simulink library "LibDBC_Some_Node_ch0_ORIGINAL"  (Simulink 9.1)
settings: Solver=VariableStepAuto  StartTime=0.0  StopTime=10.0  RelTol=1e-3
undefined symbols (not defined in the file): bit_packing, bit_unpacking, IO_Blk_Lib_TTC500, IO_CAN_ConfigMsg
libraries: IOBlock_Library_TTC580 x4, simulink x2
(part 1 of 2)
Description:
  | 10-Mai-2016 10:50:501823
settings Model: Creator=hokka  LastModifiedBy=hokka

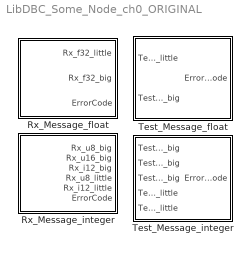
== system LibDBC_Some_Node_ch0_ORIGINAL ==
  Rx_Message_float : Subsystem  Priority=0
  Rx_Message_integer : Subsystem  Priority=0
  Test_Message_float : Subsystem  Priority=0
  Test_Message_integer : Subsystem  Priority=0

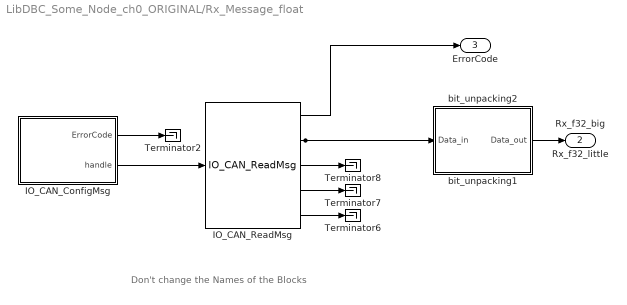
== system LibDBC_Some_Node_ch0_ORIGINAL/Rx_Message_float ==
  note: Don't change the Names of the Blocks
  IO_CAN_ConfigMsg : Subsystem  mask(IO_CAN_ConfigMsg_Code){SampleTime=-1, ttlib=IO_Blk_Lib_TTC500, ttDescription=IO_CAN_ConfigMsg, tt_iolib_version=0.19, channel=IO_CAN_CHANNEL_0, mode=IO_CAN_MSG_READ, id_format=IO_CAN_EXT_FRAME, id=0x00001021, ac_mask=0x1FFFFFFF}
      mask help: Configures a message object for the given CAN channel.
      mask init:
      | %
      mask Help: web(which('IO_CAN.h'))
      mask TypeOptions channel: IO_CAN_CHANNEL_0  | IO_CAN_CHANNEL_1 | IO_CAN_CHANNEL_2 | IO_CAN_CHANNEL_3 | IO_CAN_CHANNEL_4 | IO_CAN_CHANNEL_5 | IO_CAN_CHANNEL_6
      mask Callback channel: %
      mask TypeOptions mode: IO_CAN_MSG_READ | IO_CAN_MSG_WRITE
      mask Callback mode: %
      mask TypeOptions id_format: IO_CAN_STD_FRAME | IO_CAN_EXT_FRAME
      mask Callback id_format: %
      mask Callback id: %
      mask Callback ac_mask: %
  IO_CAN_ReadMsg : IOBlock_Library_TTC580/CAN  Blocks TTC580 IOlib/ReadMsg_CAN/IO_CAN_ReadMsg  SampleTime=-1  ttlib=IO_Blk_Lib_TTC500  ttDescription=IO_CAN_ReadMsg  tt_iolib_version=0.19
      settings: SourceProductName=I/O Blocklibrary for TTC580
  Terminator{2,6..8} (4 alike) : Terminator
  bit_unpacking1 : Subsystem  LoadFcn=|  mask(bit_unpacking_Code){SampleTime=-1, ttlib=IO_Blk_Lib_TTC500, ttDescription=bit_unpacking, tt_iolib_version=0.19, Endianness=little, Format=real32, Inversion=off, Startbit=0, Width_bits=32, Factor=1, Offset=0}
      | try
      | %
      | %Upgrade Information - standard BEGIN
      | new_color = 'blue';
      | new_ver = '0.19';
      | act_ver = get_param(gcb,'tt_iolib_version');
      | if not(strcmp(act_ver,new_ver))
      |     disp(['Upgrade block: ',gcb,char(10),'       Version: ',act_ver,' -> ',new_ver]);
      |     %switch - case for specific upgrade information e.g. additional parameter required 
      |     %Change appearance and version information
      |     set_param(gcb,'ForegroundColor',new_color);
      |     set_param(gcb,'tt_iolib_version',new_ver);
      | end
      | %Upgrade Information - standard END
      | catch
      | %Standard catch section BEGIN 
      | disp(' ');
      | disp('------------------------------------------------------------');
      | disp('An error occurred in a callback of the TTC580-BlockLib.');
      | disp(['Please check the parameters in the mask of ',gcb]);
      | disp('If you do not encounter any violations, then please '); 
      | disp('copy the following lines and report this to support@ttcontrol.com ');
      | disp('<< begin of error message dump >>');
      | disp(['Version of TTC580-BlockLib: ', get_param(gcb,'tt_iolib_version')]);
      | disp(get_param(gcb,'ttDescription'));
      | disp(gcb);
      | x=lasterror;disp(x.message);
      | disp(get_param(gcb,'MaskValues'));
      | disp(version);
      | disp(computer);
      | disp('<< end of error message dump >>');
      | disp('------------------------------------------------------------');
      | disp(' ');
      | %Standard catch section END
      | end
      mask help:
      | Block to read in CAN signal from a specified position within 64bit field.
      | For "Factor" and "Offset" the definition of Vector's CANdb applies:
      | [Physical value] = ( [Raw value] * [Factor] ) + [Offset]
      | with Raw value of a signal being the value as it is transmitted in the CAN-network
      mask init:
      | %
      mask Help: web(which('IOLib500_utils.h'))
      mask TypeOptions Endianness: big | little
      mask Callback Endianness: %
      mask TypeOptions Format: unsigned | signed | real32
      mask Callback Format: %
      mask Callback Inversion: %
      mask Callback Startbit: %
      mask Callback Width_bits: %
      mask Callback Factor: %
      mask Callback Offset: %
  bit_unpacking2 : Subsystem  LoadFcn=|  mask(bit_unpacking_Code){SampleTime=-1, ttlib=IO_Blk_Lib_TTC500, ttDescription=bit_unpacking, tt_iolib_version=0.19, Endianness=big, Format=real32, Inversion=off, Startbit=56, Width_bits=32, Factor=1, Offset=0}
      | try
      | %
      | %Upgrade Information - standard BEGIN
      | new_color = 'blue';
      | new_ver = '0.19';
      | act_ver = get_param(gcb,'tt_iolib_version');
      | if not(strcmp(act_ver,new_ver))
      |     disp(['Upgrade block: ',gcb,char(10),'       Version: ',act_ver,' -> ',new_ver]);
      |     %switch - case for specific upgrade information e.g. additional parameter required 
      |     %Change appearance and version information
      |     set_param(gcb,'ForegroundColor',new_color);
      |     set_param(gcb,'tt_iolib_version',new_ver);
      | end
      | %Upgrade Information - standard END
      | catch
      | %Standard catch section BEGIN 
      | disp(' ');
      | disp('------------------------------------------------------------');
      | disp('An error occurred in a callback of the TTC580-BlockLib.');
      | disp(['Please check the parameters in the mask of ',gcb]);
      | disp('If you do not encounter any violations, then please '); 
      | disp('copy the following lines and report this to support@ttcontrol.com ');
      | disp('<< begin of error message dump >>');
      | disp(['Version of TTC580-BlockLib: ', get_param(gcb,'tt_iolib_version')]);
      | disp(get_param(gcb,'ttDescription'));
      | disp(gcb);
      | x=lasterror;disp(x.message);
      | disp(get_param(gcb,'MaskValues'));
      | disp(version);
      | disp(computer);
      | disp('<< end of error message dump >>');
      | disp('------------------------------------------------------------');
      | disp(' ');
      | %Standard catch section END
      | end
      mask help:
      | Block to read in CAN signal from a specified position within 64bit field.
      | For "Factor" and "Offset" the definition of Vector's CANdb applies:
      | [Physical value] = ( [Raw value] * [Factor] ) + [Offset]
      | with Raw value of a signal being the value as it is transmitted in the CAN-network
      mask init:
      | %
      mask Help: web(which('IOLib500_utils.h'))
      mask TypeOptions Endianness: big | little
      mask Callback Endianness: %
      mask TypeOptions Format: unsigned | signed | real32
      mask Callback Format: %
      mask Callback Inversion: %
      mask Callback Startbit: %
      mask Callback Width_bits: %
      mask Callback Factor: %
      mask Callback Offset: %
  Rx_f32_little : Outport
  Rx_f32_big : Outport  Port=2
  ErrorCode : Outport  Port=3
  wires:
  IO_CAN_ReadMsg/3 -> Terminator8/1
  IO_CAN_ReadMsg/4 -> Terminator7/1
  IO_CAN_ReadMsg/5 -> Terminator6/1
  IO_CAN_ConfigMsg/2(handle) -> IO_CAN_ReadMsg/1
  IO_CAN_ConfigMsg/1(ErrorCode) -> Terminator2/1
  IO_CAN_ReadMsg/1 -> ErrorCode/1
  IO_CAN_ReadMsg/2 -> bit_unpacking1/1(Data_in), bit_unpacking2/1(Data_in)
  bit_unpacking1/1(Data_out) -> Rx_f32_little/1
  bit_unpacking2/1(Data_out) -> Rx_f32_big/1

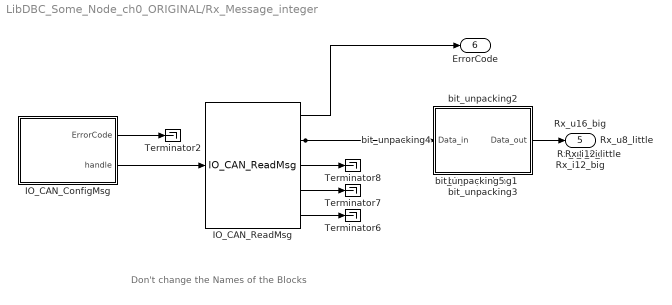
== system LibDBC_Some_Node_ch0_ORIGINAL/Rx_Message_integer ==
  note: Don't change the Names of the Blocks
  IO_CAN_ConfigMsg : Subsystem  mask(IO_CAN_ConfigMsg_Code){SampleTime=-1, ttlib=IO_Blk_Lib_TTC500, ttDescription=IO_CAN_ConfigMsg, tt_iolib_version=0.19, channel=IO_CAN_CHANNEL_0, mode=IO_CAN_MSG_READ, id_format=IO_CAN_STD_FRAME, id=0x020, ac_mask=0x7FF}
      mask help: Configures a message object for the given CAN channel.
      mask init:
      | %
      mask Help: web(which('IO_CAN.h'))
      mask TypeOptions channel: IO_CAN_CHANNEL_0  | IO_CAN_CHANNEL_1 | IO_CAN_CHANNEL_2 | IO_CAN_CHANNEL_3 | IO_CAN_CHANNEL_4 | IO_CAN_CHANNEL_5 | IO_CAN_CHANNEL_6
      mask Callback channel: %
      mask TypeOptions mode: IO_CAN_MSG_READ | IO_CAN_MSG_WRITE
      mask Callback mode: %
      mask TypeOptions id_format: IO_CAN_STD_FRAME | IO_CAN_EXT_FRAME
      mask Callback id_format: %
      mask Callback id: %
      mask Callback ac_mask: %
  IO_CAN_ReadMsg : IOBlock_Library_TTC580/CAN  Blocks TTC580 IOlib/ReadMsg_CAN/IO_CAN_ReadMsg  SampleTime=-1  ttlib=IO_Blk_Lib_TTC500  ttDescription=IO_CAN_ReadMsg  tt_iolib_version=0.19
      settings: SourceProductName=I/O Blocklibrary for TTC580
  Terminator{2,6..8} (4 alike) : Terminator
  bit_unpacking1 : Subsystem  LoadFcn=|  mask(bit_unpacking_Code){SampleTime=-1, ttlib=IO_Blk_Lib_TTC500, ttDescription=bit_unpacking, tt_iolib_version=0.19, Endianness=big, Format=unsigned, Inversion=off, Startbit=0, Width_bits=8, Factor=1, Offset=0}
      | try
      | %
      | %Upgrade Information - standard BEGIN
      | new_color = 'blue';
      | new_ver = '0.19';
      | act_ver = get_param(gcb,'tt_iolib_version');
      | if not(strcmp(act_ver,new_ver))
      |     disp(['Upgrade block: ',gcb,char(10),'       Version: ',act_ver,' -> ',new_ver]);
      |     %switch - case for specific upgrade information e.g. additional parameter required 
      |     %Change appearance and version information
      |     set_param(gcb,'ForegroundColor',new_color);
      |     set_param(gcb,'tt_iolib_version',new_ver);
      | end
      | %Upgrade Information - standard END
      | catch
      | %Standard catch section BEGIN 
      | disp(' ');
      | disp('------------------------------------------------------------');
      | disp('An error occurred in a callback of the TTC580-BlockLib.');
      | disp(['Please check the parameters in the mask of ',gcb]);
      | disp('If you do not encounter any violations, then please '); 
      | disp('copy the following lines and report this to support@ttcontrol.com ');
      | disp('<< begin of error message dump >>');
      | disp(['Version of TTC580-BlockLib: ', get_param(gcb,'tt_iolib_version')]);
      | disp(get_param(gcb,'ttDescription'));
      | disp(gcb);
      | x=lasterror;disp(x.message);
      | disp(get_param(gcb,'MaskValues'));
      | disp(version);
      | disp(computer);
      | disp('<< end of error message dump >>');
      | disp('------------------------------------------------------------');
      | disp(' ');
      | %Standard catch section END
      | end
      mask help:
      | Block to read in CAN signal from a specified position within 64bit field.
      | For "Factor" and "Offset" the definition of Vector's CANdb applies:
      | [Physical value] = ( [Raw value] * [Factor] ) + [Offset]
      | with Raw value of a signal being the value as it is transmitted in the CAN-network
      mask init:
      | %
      mask Help: web(which('IOLib500_utils.h'))
      mask TypeOptions Endianness: big | little
      mask Callback Endianness: %
      mask TypeOptions Format: unsigned | signed | real32
      mask Callback Format: %
      mask Callback Inversion: %
      mask Callback Startbit: %
      mask Callback Width_bits: %
      mask Callback Factor: %
      mask Callback Offset: %
  bit_unpacking2 : Subsystem  LoadFcn=|  mask(bit_unpacking_Code){SampleTime=-1, ttlib=IO_Blk_Lib_TTC500, ttDescription=bit_unpacking, tt_iolib_version=0.19, Endianness=big, Format=unsigned, Inversion=off, Startbit=16, Width_bits=16, Factor=1, Offset=0}
      | try
      | %
      | %Upgrade Information - standard BEGIN
      | new_color = 'blue';
      | new_ver = '0.19';
      | act_ver = get_param(gcb,'tt_iolib_version');
      | if not(strcmp(act_ver,new_ver))
      |     disp(['Upgrade block: ',gcb,char(10),'       Version: ',act_ver,' -> ',new_ver]);
      |     %switch - case for specific upgrade information e.g. additional parameter required 
      |     %Change appearance and version information
      |     set_param(gcb,'ForegroundColor',new_color);
      |     set_param(gcb,'tt_iolib_version',new_ver);
      | end
      | %Upgrade Information - standard END
      | catch
      | %Standard catch section BEGIN 
      | disp(' ');
      | disp('------------------------------------------------------------');
      | disp('An error occurred in a callback of the TTC580-BlockLib.');
      | disp(['Please check the parameters in the mask of ',gcb]);
      | disp('If you do not encounter any violations, then please '); 
      | disp('copy the following lines and report this to support@ttcontrol.com ');
      | disp('<< begin of error message dump >>');
      | disp(['Version of TTC580-BlockLib: ', get_param(gcb,'tt_iolib_version')]);
      | disp(get_param(gcb,'ttDescription'));
      | disp(gcb);
      | x=lasterror;disp(x.message);
      | disp(get_param(gcb,'MaskValues'));
      | disp(version);
      | disp(computer);
      | disp('<< end of error message dump >>');
      | disp('------------------------------------------------------------');
      | disp(' ');
      | %Standard catch section END
      | end
      mask help:
      | Block to read in CAN signal from a specified position within 64bit field.
      | For "Factor" and "Offset" the definition of Vector's CANdb applies:
      | [Physical value] = ( [Raw value] * [Factor] ) + [Offset]
      | with Raw value of a signal being the value as it is transmitted in the CAN-network
      mask init:
      | %
      mask Help: web(which('IOLib500_utils.h'))
      mask TypeOptions Endianness: big | little
      mask Callback Endianness: %
      mask TypeOptions Format: unsigned | signed | real32
      mask Callback Format: %
      mask Callback Inversion: %
      mask Callback Startbit: %
      mask Callback Width_bits: %
      mask Callback Factor: %
      mask Callback Offset: %
  bit_unpacking3 : Subsystem  LoadFcn=|  mask(bit_unpacking_Code){SampleTime=-1, ttlib=IO_Blk_Lib_TTC500, ttDescription=bit_unpacking, tt_iolib_version=0.19, Endianness=big, Format=signed, Inversion=off, Startbit=35, Width_bits=12, Factor=1, Offset=0}
      | try
      | %
      | %Upgrade Information - standard BEGIN
      | new_color = 'blue';
      | new_ver = '0.19';
      | act_ver = get_param(gcb,'tt_iolib_version');
      | if not(strcmp(act_ver,new_ver))
      |     disp(['Upgrade block: ',gcb,char(10),'       Version: ',act_ver,' -> ',new_ver]);
      |     %switch - case for specific upgrade information e.g. additional parameter required 
      |     %Change appearance and version information
      |     set_param(gcb,'ForegroundColor',new_color);
      |     set_param(gcb,'tt_iolib_version',new_ver);
      | end
      | %Upgrade Information - standard END
      | catch
      | %Standard catch section BEGIN 
      | disp(' ');
      | disp('------------------------------------------------------------');
      | disp('An error occurred in a callback of the TTC580-BlockLib.');
      | disp(['Please check the parameters in the mask of ',gcb]);
      | disp('If you do not encounter any violations, then please '); 
      | disp('copy the following lines and report this to support@ttcontrol.com ');
      | disp('<< begin of error message dump >>');
      | disp(['Version of TTC580-BlockLib: ', get_param(gcb,'tt_iolib_version')]);
      | disp(get_param(gcb,'ttDescription'));
      | disp(gcb);
      | x=lasterror;disp(x.message);
      | disp(get_param(gcb,'MaskValues'));
      | disp(version);
      | disp(computer);
      | disp('<< end of error message dump >>');
      | disp('------------------------------------------------------------');
      | disp(' ');
      | %Standard catch section END
      | end
      mask help:
      | Block to read in CAN signal from a specified position within 64bit field.
      | For "Factor" and "Offset" the definition of Vector's CANdb applies:
      | [Physical value] = ( [Raw value] * [Factor] ) + [Offset]
      | with Raw value of a signal being the value as it is transmitted in the CAN-network
      mask init:
      | %
      mask Help: web(which('IOLib500_utils.h'))
      mask TypeOptions Endianness: big | little
      mask Callback Endianness: %
      mask TypeOptions Format: unsigned | signed | real32
      mask Callback Format: %
      mask Callback Inversion: %
      mask Callback Startbit: %
      mask Callback Width_bits: %
      mask Callback Factor: %
      mask Callback Offset: %
  bit_unpacking4 : Subsystem  LoadFcn=|  mask(bit_unpacking_Code){SampleTime=-1, ttlib=IO_Blk_Lib_TTC500, ttDescription=bit_unpacking, tt_iolib_version=0.19, Endianness=little, Format=unsigned, Inversion=off, Startbit=40, Width_bits=8, Factor=1, Offset=0}
      | try
      | %
      | %Upgrade Information - standard BEGIN
      | new_color = 'blue';
      | new_ver = '0.19';
      | act_ver = get_param(gcb,'tt_iolib_version');
      | if not(strcmp(act_ver,new_ver))
      |     disp(['Upgrade block: ',gcb,char(10),'       Version: ',act_ver,' -> ',new_ver]);
      |     %switch - case for specific upgrade information e.g. additional parameter required 
      |     %Change appearance and version information
      |     set_param(gcb,'ForegroundColor',new_color);
      |     set_param(gcb,'tt_iolib_version',new_ver);
      | end
      | %Upgrade Information - standard END
      | catch
      | %Standard catch section BEGIN 
      | disp(' ');
      | disp('------------------------------------------------------------');
      | disp('An error occurred in a callback of the TTC580-BlockLib.');
      | disp(['Please check the parameters in the mask of ',gcb]);
      | disp('If you do not encounter any violations, then please '); 
      | disp('copy the following lines and report this to support@ttcontrol.com ');
      | disp('<< begin of error message dump >>');
      | disp(['Version of TTC580-BlockLib: ', get_param(gcb,'tt_iolib_version')]);
      | disp(get_param(gcb,'ttDescription'));
      | disp(gcb);
      | x=lasterror;disp(x.message);
      | disp(get_param(gcb,'MaskValues'));
      | disp(version);
      | disp(computer);
      | disp('<< end of error message dump >>');
      | disp('------------------------------------------------------------');
      | disp(' ');
      | %Standard catch section END
      | end
      mask help:
      | Block to read in CAN signal from a specified position within 64bit field.
      | For "Factor" and "Offset" the definition of Vector's CANdb applies:
      | [Physical value] = ( [Raw value] * [Factor] ) + [Offset]
      | with Raw value of a signal being the value as it is transmitted in the CAN-network
      mask init:
      | %
      mask Help: web(which('IOLib500_utils.h'))
      mask TypeOptions Endianness: big | little
      mask Callback Endianness: %
      mask TypeOptions Format: unsigned | signed | real32
      mask Callback Format: %
      mask Callback Inversion: %
      mask Callback Startbit: %
      mask Callback Width_bits: %
      mask Callback Factor: %
      mask Callback Offset: %
  bit_unpacking5 : Subsystem  LoadFcn=|  mask(bit_unpacking_Code){SampleTime=-1, ttlib=IO_Blk_Lib_TTC500, ttDescription=bit_unpacking, tt_iolib_version=0.19, Endianness=little, Format=signed, Inversion=off, Startbit=49, Width_bits=12, Factor=1, Offset=0}
      | try
      | %
      | %Upgrade Information - standard BEGIN
      | new_color = 'blue';
      | new_ver = '0.19';
      | act_ver = get_param(gcb,'tt_iolib_version');
      | if not(strcmp(act_ver,new_ver))
      |     disp(['Upgrade block: ',gcb,char(10),'       Version: ',act_ver,' -> ',new_ver]);
      |     %switch - case for specific upgrade information e.g. additional parameter required 
      |     %Change appearance and version information
      |     set_param(gcb,'ForegroundColor',new_color);
      |     set_param(gcb,'tt_iolib_version',new_ver);
      | end
      | %Upgrade Information - standard END
      | catch
      | %Standard catch section BEGIN 
      | disp(' ');
      | disp('------------------------------------------------------------');
      | disp('An error occurred in a callback of the TTC580-BlockLib.');
      | disp(['Please check the parameters in the mask of ',gcb]);
      | disp('If you do not encounter any violations, then please '); 
      | disp('copy the following lines and report this to support@ttcontrol.com ');
      | disp('<< begin of error message dump >>');
      | disp(['Version of TTC580-BlockLib: ', get_param(gcb,'tt_iolib_version')]);
      | disp(get_param(gcb,'ttDescription'));
      | disp(gcb);
      | x=lasterror;disp(x.message);
      | disp(get_param(gcb,'MaskValues'));
      | disp(version);
      | disp(computer);
      | disp('<< end of error message dump >>');
      | disp('------------------------------------------------------------');
      | disp(' ');
      | %Standard catch section END
      | end
      mask help:
      | Block to read in CAN signal from a specified position within 64bit field.
      | For "Factor" and "Offset" the definition of Vector's CANdb applies:
      | [Physical value] = ( [Raw value] * [Factor] ) + [Offset]
      | with Raw value of a signal being the value as it is transmitted in the CAN-network
      mask init:
      | %
      mask Help: web(which('IOLib500_utils.h'))
      mask TypeOptions Endianness: big | little
      mask Callback Endianness: %
      mask TypeOptions Format: unsigned | signed | real32
      mask Callback Format: %
      mask Callback Inversion: %
      mask Callback Startbit: %
      mask Callback Width_bits: %
      mask Callback Factor: %
      mask Callback Offset: %
  Rx_u8_big : Outport
  Rx_u16_big : Outport  Port=2
  Rx_i12_big : Outport  Port=3
  Rx_u8_little : Outport  Port=4
  Rx_i12_little : Outport  Port=5
  ErrorCode : Outport  Port=6
  wires:
  IO_CAN_ReadMsg/3 -> Terminator8/1
  IO_CAN_ReadMsg/4 -> Terminator7/1
  IO_CAN_ReadMsg/5 -> Terminator6/1
  IO_CAN_ConfigMsg/2(handle) -> IO_CAN_ReadMsg/1
  IO_CAN_ConfigMsg/1(ErrorCode) -> Terminator2/1
  IO_CAN_ReadMsg/1 -> ErrorCode/1
  IO_CAN_ReadMsg/2 -> bit_unpacking1/1(Data_in), bit_unpacking2/1(Data_in), bit_unpacking3/1(Data_in), bit_unpacking4/1(Data_in), bit_unpacking5/1(Data_in)
  bit_unpacking1/1(Data_out) -> Rx_u8_big/1
  bit_unpacking2/1(Data_out) -> Rx_u16_big/1
  bit_unpacking3/1(Data_out) -> Rx_i12_big/1
  bit_unpacking4/1(Data_out) -> Rx_u8_little/1
  bit_unpacking5/1(Data_out) -> Rx_i12_little/1

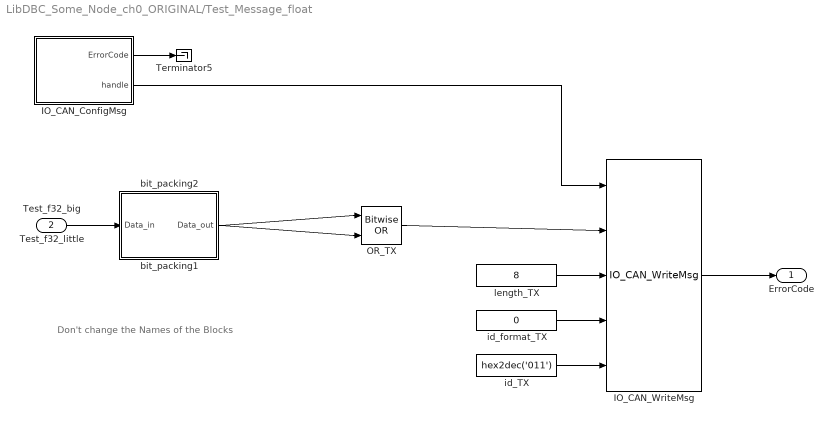
== system LibDBC_Some_Node_ch0_ORIGINAL/Test_Message_float ==
  note: Don't change the Names of the Blocks
  Test_f32_little : Inport
  Test_f32_big : Inport  Port=2
  IO_CAN_ConfigMsg : Subsystem  mask(IO_CAN_ConfigMsg_Code){SampleTime=-1, ttlib=IO_Blk_Lib_TTC500, ttDescription=IO_CAN_ConfigMsg, tt_iolib_version=0.19, channel=IO_CAN_CHANNEL_0, mode=IO_CAN_MSG_WRITE, id_format=IO_CAN_STD_FRAME, id=0x011, ac_mask=0x7FF}
      mask help: Configures a message object for the given CAN channel.
      mask init:
      | %
      mask Help: web(which('IO_CAN.h'))
      mask TypeOptions channel: IO_CAN_CHANNEL_0  | IO_CAN_CHANNEL_1 | IO_CAN_CHANNEL_2 | IO_CAN_CHANNEL_3 | IO_CAN_CHANNEL_4 | IO_CAN_CHANNEL_5 | IO_CAN_CHANNEL_6
      mask Callback channel: %
      mask TypeOptions mode: IO_CAN_MSG_READ | IO_CAN_MSG_WRITE
      mask Callback mode: %
      mask TypeOptions id_format: IO_CAN_STD_FRAME | IO_CAN_EXT_FRAME
      mask Callback id_format: %
      mask Callback id: %
      mask Callback ac_mask: %
  IO_CAN_WriteMsg : IOBlock_Library_TTC580/CAN  Blocks TTC580 IOlib/WriteMsg_CAN/IO_CAN_WriteMsg  SampleTime=-1  ttlib=IO_Blk_Lib_TTC500  ttDescription=IO_CAN_WriteMsg  tt_iolib_version=0.19
      settings: SourceProductName=I/O Blocklibrary for TTC580
  OR_TX : simulink/Logic and Bit Operations/Bitwise Operator  logicop=OR  UseBitMask=off  NumInputPorts=2  BitMask=bin2dec('11011001')  BitMaskRealWorld=Stored Integer
  Terminator5 : Terminator
  bit_packing1 : Subsystem  LoadFcn=|  mask(bit_packing_Code){SampleTime=-1, ttlib=IO_Blk_Lib_TTC500, ttDescription=bit_packing, tt_iolib_version=0.19, Endianness=little, Format=real32, Inversion=off, Startbit=0, Width_bits=32, Factor=1, Offset=0}
      | try
      | %
      | %Upgrade Information - standard BEGIN
      | new_color = 'blue';
      | new_ver = '0.19';
      | act_ver = get_param(gcb,'tt_iolib_version');
      | if not(strcmp(act_ver,new_ver))
      |     disp(['Upgrade block: ',gcb,char(10),'       Version: ',act_ver,' -> ',new_ver]);
      |     %switch - case for specific upgrade information e.g. additional parameter required 
      |     %Change appearance and version information
      |     set_param(gcb,'ForegroundColor',new_color);
      |     set_param(gcb,'tt_iolib_version',new_ver);
      | end
      | %Upgrade Information - standard END
      | catch
      | %Standard catch section BEGIN 
      | disp(' ');
      | disp('------------------------------------------------------------');
      | disp('An error occurred in a callback of the TTC580-BlockLib.');
      | disp(['Please check the parameters in the mask of ',gcb]);
      | disp('If you do not encounter any violations, then please '); 
      | disp('copy the following lines and report this to support@ttcontrol.com ');
      | disp('<< begin of error message dump >>');
      | disp(['Version of TTC580-BlockLib: ', get_param(gcb,'tt_iolib_version')]);
      | disp(get_param(gcb,'ttDescription'));
      | disp(gcb);
      | x=lasterror;disp(x.message);
      | disp(get_param(gcb,'MaskValues'));
      | disp(version);
      | disp(computer);
      | disp('<< end of error message dump >>');
      | disp('------------------------------------------------------------');
      | disp(' ');
      | %Standard catch section END
      | end
      mask help:
      | Block to prepare CAN-transmition at specified position within 64bit field.
      | For "Factor" and "Offset" the definition of Vector's CANdb applies:
      | [Physical value] = ( [Raw value] * [Factor] ) + [Offset]
      | with Raw value of a signal being the value as it is transmitted in the CAN-network.
      mask init:
      | %
      mask Help: web(which('IOLib500_utils.h'))
      mask TypeOptions Endianness: big | little
      mask Callback Endianness: %
      mask TypeOptions Format: unsigned | signed | real32
      mask Callback Format: %
      mask Callback Inversion: %
      mask Callback Startbit: %
      mask Callback Width_bits: %
      mask Callback Factor: %
      mask Callback Offset: %
  bit_packing2 : Subsystem  LoadFcn=|  mask(bit_packing_Code){SampleTime=-1, ttlib=IO_Blk_Lib_TTC500, ttDescription=bit_packing, tt_iolib_version=0.19, Endianness=big, Format=real32, Inversion=off, Startbit=56, Width_bits=32, Factor=1, Offset=0}
      | try
      | %
      | %Upgrade Information - standard BEGIN
      | new_color = 'blue';
      | new_ver = '0.19';
      | act_ver = get_param(gcb,'tt_iolib_version');
      | if not(strcmp(act_ver,new_ver))
      |     disp(['Upgrade block: ',gcb,char(10),'       Version: ',act_ver,' -> ',new_ver]);
      |     %switch - case for specific upgrade information e.g. additional parameter required 
      |     %Change appearance and version information
      |     set_param(gcb,'ForegroundColor',new_color);
      |     set_param(gcb,'tt_iolib_version',new_ver);
      | end
      | %Upgrade Information - standard END
      | catch
      | %Standard catch section BEGIN 
      | disp(' ');
      | disp('------------------------------------------------------------');
      | disp('An error occurred in a callback of the TTC580-BlockLib.');
      | disp(['Please check the parameters in the mask of ',gcb]);
      | disp('If you do not encounter any violations, then please '); 
      | disp('copy the following lines and report this to support@ttcontrol.com ');
      | disp('<< begin of error message dump >>');
      | disp(['Version of TTC580-BlockLib: ', get_param(gcb,'tt_iolib_version')]);
      | disp(get_param(gcb,'ttDescription'));
      | disp(gcb);
      | x=lasterror;disp(x.message);
      | disp(get_param(gcb,'MaskValues'));
      | disp(version);
      | disp(computer);
      | disp('<< end of error message dump >>');
      | disp('------------------------------------------------------------');
      | disp(' ');
      | %Standard catch section END
      | end
      mask help:
      | Block to prepare CAN-transmition at specified position within 64bit field.
      | For "Factor" and "Offset" the definition of Vector's CANdb applies:
      | [Physical value] = ( [Raw value] * [Factor] ) + [Offset]
      | with Raw value of a signal being the value as it is transmitted in the CAN-network.
      mask init:
      | %
      mask Help: web(which('IOLib500_utils.h'))
      mask TypeOptions Endianness: big | little
      mask Callback Endianness: %
      mask TypeOptions Format: unsigned | signed | real32
      mask Callback Format: %
      mask Callback Inversion: %
      mask Callback Startbit: %
      mask Callback Width_bits: %
      mask Callback Factor: %
      mask Callback Offset: %
  id_TX : Constant  Value=hex2dec('011')  OutDataTypeStr=uint32
  id_format_TX : Constant  Value=0  OutDataTypeStr=Inherit: Inherit via back propagation
  length_TX : Constant  Value=8  OutDataTypeStr=Inherit: Inherit via back propagation
  ErrorCode : Outport
  wires:
  id_TX/1 -> IO_CAN_WriteMsg/5
  id_format_TX/1 -> IO_CAN_WriteMsg/4
  length_TX/1 -> IO_CAN_WriteMsg/3
  IO_CAN_ConfigMsg/2(handle) -> IO_CAN_WriteMsg/1
  IO_CAN_ConfigMsg/1(ErrorCode) -> Terminator5/1
  IO_CAN_WriteMsg/1 -> ErrorCode/1
  Test_f32_little/1 -> bit_packing1/1(Data_in)
  bit_packing1/1(Data_out) -> OR_TX/1
  Test_f32_big/1 -> bit_packing2/1(Data_in)
  bit_packing2/1(Data_out) -> OR_TX/2
  OR_TX/1 -> IO_CAN_WriteMsg/2

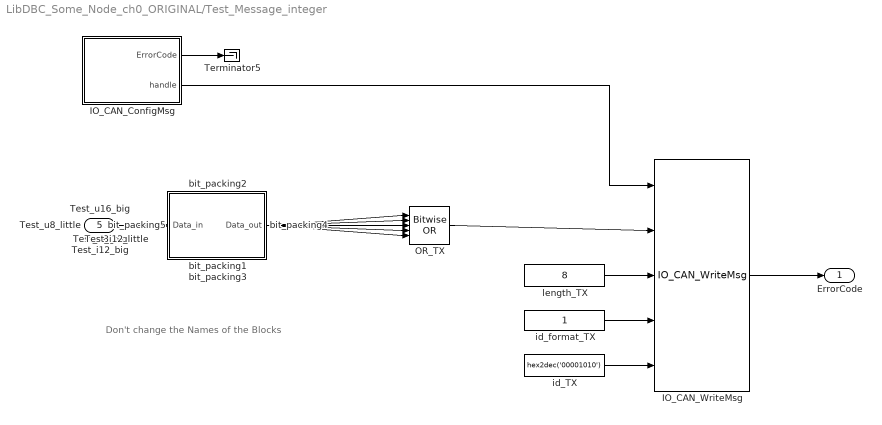
== system LibDBC_Some_Node_ch0_ORIGINAL/Test_Message_integer ==
  note: Don't change the Names of the Blocks
  Test_u8_big : Inport
  Test_u16_big : Inport  Port=2
  Test_i12_big : Inport  Port=3
  Test_u8_little : Inport  Port=4
  Test_i12_little : Inport  Port=5
  IO_CAN_ConfigMsg : Subsystem  mask(IO_CAN_ConfigMsg_Code){SampleTime=-1, ttlib=IO_Blk_Lib_TTC500, ttDescription=IO_CAN_ConfigMsg, tt_iolib_version=0.19, channel=IO_CAN_CHANNEL_0, mode=IO_CAN_MSG_WRITE, id_format=IO_CAN_EXT_FRAME, id=0x00001010, ac_mask=0x1FFFFFFF}
      mask help: Configures a message object for the given CAN channel.
      mask init:
      | %
      mask Help: web(which('IO_CAN.h'))
      mask TypeOptions channel: IO_CAN_CHANNEL_0  | IO_CAN_CHANNEL_1 | IO_CAN_CHANNEL_2 | IO_CAN_CHANNEL_3 | IO_CAN_CHANNEL_4 | IO_CAN_CHANNEL_5 | IO_CAN_CHANNEL_6
      mask Callback channel: %
      mask TypeOptions mode: IO_CAN_MSG_READ | IO_CAN_MSG_WRITE
      mask Callback mode: %
      mask TypeOptions id_format: IO_CAN_STD_FRAME | IO_CAN_EXT_FRAME
      mask Callback id_format: %
      mask Callback id: %
      mask Callback ac_mask: %
  IO_CAN_WriteMsg : IOBlock_Library_TTC580/CAN  Blocks TTC580 IOlib/WriteMsg_CAN/IO_CAN_WriteMsg  SampleTime=-1  ttlib=IO_Blk_Lib_TTC500  ttDescription=IO_CAN_WriteMsg  tt_iolib_version=0.19
      settings: SourceProductName=I/O Blocklibrary for TTC580
  OR_TX : simulink/Logic and Bit Operations/Bitwise Operator  logicop=OR  UseBitMask=off  NumInputPorts=5  BitMask=bin2dec('11011001')  BitMaskRealWorld=Stored Integer
  Terminator5 : Terminator
  bit_packing1 : Subsystem  LoadFcn=|  mask(bit_packing_Code){SampleTime=-1, ttlib=IO_Blk_Lib_TTC500, ttDescription=bit_packing, tt_iolib_version=0.19, Endianness=big, Format=unsigned, Inversion=off, Startbit=13, Width_bits=8, Factor=1, Offset=0}
      | try
      | %
      | %Upgrade Information - standard BEGIN
      | new_color = 'blue';
      | new_ver = '0.19';
      | act_ver = get_param(gcb,'tt_iolib_version');
      | if not(strcmp(act_ver,new_ver))
      |     disp(['Upgrade block: ',gcb,char(10),'       Version: ',act_ver,' -> ',new_ver]);
      |     %switch - case for specific upgrade information e.g. additional parameter required 
      |     %Change appearance and version information
      |     set_param(gcb,'ForegroundColor',new_color);
      |     set_param(gcb,'tt_iolib_version',new_ver);
      | end
      | %Upgrade Information - standard END
      | catch
      | %Standard catch section BEGIN 
      | disp(' ');
      | disp('------------------------------------------------------------');
      | disp('An error occurred in a callback of the TTC580-BlockLib.');
      | disp(['Please check the parameters in the mask of ',gcb]);
      | disp('If you do not encounter any violations, then please '); 
      | disp('copy the following lines and report this to support@ttcontrol.com ');
      | disp('<< begin of error message dump >>');
      | disp(['Version of TTC580-BlockLib: ', get_param(gcb,'tt_iolib_version')]);
      | disp(get_param(gcb,'ttDescription'));
      | disp(gcb);
      | x=lasterror;disp(x.message);
      | disp(get_param(gcb,'MaskValues'));
      | disp(version);
      | disp(computer);
      | disp('<< end of error message dump >>');
      | disp('------------------------------------------------------------');
      | disp(' ');
      | %Standard catch section END
      | end
      mask help:
      | Block to prepare CAN-transmition at specified position within 64bit field.
      | For "Factor" and "Offset" the definition of Vector's CANdb applies:
      | [Physical value] = ( [Raw value] * [Factor] ) + [Offset]
      | with Raw value of a signal being the value as it is transmitted in the CAN-network.
      mask init:
      | %
      mask Help: web(which('IOLib500_utils.h'))
      mask TypeOptions Endianness: big | little
      mask Callback Endianness: %
      mask TypeOptions Format: unsigned | signed | real32
      mask Callback Format: %
      mask Callback Inversion: %
      mask Callback Startbit: %
      mask Callback Width_bits: %
      mask Callback Factor: %
      mask Callback Offset: %
  bit_packing2 : Subsystem  LoadFcn=|  mask(bit_packing_Code){SampleTime=-1, ttlib=IO_Blk_Lib_TTC500, ttDescription=bit_packing, tt_iolib_version=0.19, Endianness=big, Format=unsigned, Inversion=off, Startbit=29, Width_bits=16, Factor=1, Offset=0}
      | try
      | %
      | %Upgrade Information - standard BEGIN
      | new_color = 'blue';
      | new_ver = '0.19';
      | act_ver = get_param(gcb,'tt_iolib_version');
      | if not(strcmp(act_ver,new_ver))
      |     disp(['Upgrade block: ',gcb,char(10),'       Version: ',act_ver,' -> ',new_ver]);
      |     %switch - case for specific upgrade information e.g. additional parameter required 
      |     %Change appearance and version information
      |     set_param(gcb,'ForegroundColor',new_color);
      |     set_param(gcb,'tt_iolib_version',new_ver);
      | end
      | %Upgrade Information - standard END
      | catch
      | %Standard catch section BEGIN 
      | disp(' ');
      | disp('------------------------------------------------------------');
      | disp('An error occurred in a callback of the TTC580-BlockLib.');
      | disp(['Please check the parameters in the mask of ',gcb]);
      | disp('If you do not encounter any violations, then please '); 
      | disp('copy the following lines and report this to support@ttcontrol.com ');
      | disp('<< begin of error message dump >>');
      | disp(['Version of TTC580-BlockLib: ', get_param(gcb,'tt_iolib_version')]);
      | disp(get_param(gcb,'ttDescription'));
      | disp(gcb);
      | x=lasterror;disp(x.message);
      | disp(get_param(gcb,'MaskValues'));
      | disp(version);
      | disp(computer);
      | disp('<< end of error message dump >>');
      | disp('------------------------------------------------------------');
      | disp(' ');
      | %Standard catch section END
      | end
      mask help:
      | Block to prepare CAN-transmition at specified position within 64bit field.
      | For "Factor" and "Offset" the definition of Vector's CANdb applies:
      | [Physical value] = ( [Raw value] * [Factor] ) + [Offset]
      | with Raw value of a signal being the value as it is transmitted in the CAN-network.
      mask init:
      | %
      mask Help: web(which('IOLib500_utils.h'))
      mask TypeOptions Endianness: big | little
      mask Callback Endianness: %
      mask TypeOptions Format: unsigned | signed | real32
      mask Callback Format: %
      mask Callback Inversion: %
      mask Callback Startbit: %
      mask Callback Width_bits: %
      mask Callback Factor: %
      mask Callback Offset: %
  bit_packing3 : Subsystem  LoadFcn=|  mask(bit_packing_Code){SampleTime=-1, ttlib=IO_Blk_Lib_TTC500, ttDescription=bit_packing, tt_iolib_version=0.19, Endianness=big, Format=signed, Inversion=off, Startbit=33, Width_bits=12, Factor=1, Offset=0}
      | try
      | %
      | %Upgrade Information - standard BEGIN
      | new_color = 'blue';
      | new_ver = '0.19';
      | act_ver = get_param(gcb,'tt_iolib_version');
      | if not(strcmp(act_ver,new_ver))
      |     disp(['Upgrade block: ',gcb,char(10),'       Version: ',act_ver,' -> ',new_ver]);
      |     %switch - case for specific upgrade information e.g. additional parameter required 
      |     %Change appearance and version information
      |     set_param(gcb,'ForegroundColor',new_color);
      |     set_param(gcb,'tt_iolib_version',new_ver);
      | end
      | %Upgrade Information - standard END
      | catch
      | %Standard catch section BEGIN 
      | disp(' ');
      | disp('------------------------------------------------------------');
      | disp('An error occurred in a callback of the TTC580-BlockLib.');
      | disp(['Please check the parameters in the mask of ',gcb]);
      | disp('If you do not encounter any violations, then please '); 
      | disp('copy the following lines and report this to support@ttcontrol.com ');
      | disp('<< begin of error message dump >>');
      | disp(['Version of TTC580-BlockLib: ', get_param(gcb,'tt_iolib_version')]);
      | disp(get_param(gcb,'ttDescription'));
      | disp(gcb);
      | x=lasterror;disp(x.message);
      | disp(get_param(gcb,'MaskValues'));
      | disp(version);
      | disp(computer);
      | disp('<< end of error message dump >>');
      | disp('------------------------------------------------------------');
      | disp(' ');
      | %Standard catch section END
      | end
      mask help:
      | Block to prepare CAN-transmition at specified position within 64bit field.
      | For "Factor" and "Offset" the definition of Vector's CANdb applies:
      | [Physical value] = ( [Raw value] * [Factor] ) + [Offset]
      | with Raw value of a signal being the value as it is transmitted in the CAN-network.
      mask init:
      | %
      mask Help: web(which('IOLib500_utils.h'))
      mask TypeOptions Endianness: big | little
      mask Callback Endianness: %
      mask TypeOptions Format: unsigned | signed | real32
      mask Callback Format: %
      mask Callback Inversion: %
      mask Callback Startbit: %
      mask Callback Width_bits: %
      mask Callback Factor: %
      mask Callback Offset: %
  bit_packing4 : Subsystem  LoadFcn=|  mask(bit_packing_Code){SampleTime=-1, ttlib=IO_Blk_Lib_TTC500, ttDescription=bit_packing, tt_iolib_version=0.19, Endianness=little, Format=unsigned, Inversion=off, Startbit=42, Width_bits=8, Factor=1, Offset=0}
      | try
      | %
      | %Upgrade Information - standard BEGIN
      | new_color = 'blue';
      | new_ver = '0.19';
      | act_ver = get_param(gcb,'tt_iolib_version');
      | if not(strcmp(act_ver,new_ver))
      |     disp(['Upgrade block: ',gcb,char(10),'       Version: ',act_ver,' -> ',new_ver]);
      |     %switch - case for specific upgrade information e.g. additional parameter required 
      |     %Change appearance and version information
      |     set_param(gcb,'ForegroundColor',new_color);
      |     set_param(gcb,'tt_iolib_version',new_ver);
      | end
      | %Upgrade Information - standard END
      | catch
      | %Standard catch section BEGIN 
      | disp(' ');
      | disp('------------------------------------------------------------');
      | disp('An error occurred in a callback of the TTC580-BlockLib.');
      | disp(['Please check the parameters in the mask of ',gcb]);
      | disp('If you do not encounter any violations, then please '); 
      | disp('copy the following lines and report this to support@ttcontrol.com ');
      | disp('<< begin of error message dump >>');
      | disp(['Version of TTC580-BlockLib: ', get_param(gcb,'tt_iolib_version')]);
      | disp(get_param(gcb,'ttDescription'));
      | disp(gcb);
      | x=lasterror;disp(x.message);
      | disp(get_param(gcb,'MaskValues'));
      | disp(version);
      | disp(computer);
      | disp('<< end of error message dump >>');
      | disp('------------------------------------------------------------');
      | disp(' ');
      | %Standard catch section END
      | end
      mask help:
      | Block to prepare CAN-transmition at specified position within 64bit field.
      | For "Factor" and "Offset" the definition of Vector's CANdb applies:
      | [Physical value] = ( [Raw value] * [Factor] ) + [Offset]
      | with Raw value of a signal being the value as it is transmitted in the CAN-network.
      mask init:
      | %
      mask Help: web(which('IOLib500_utils.h'))
      mask TypeOptions Endianness: big | little
      mask Callback Endianness: %
      mask TypeOptions Format: unsigned | signed | real32
      mask Callback Format: %
      mask Callback Inversion: %
      mask Callback Startbit: %
      mask Callback Width_bits: %
      mask Callback Factor: %
      mask Callback Offset: %
  bit_packing5 : Subsystem  LoadFcn=|  mask(bit_packing_Code){SampleTime=-1, ttlib=IO_Blk_Lib_TTC500, ttDescription=bit_packing, tt_iolib_version=0.19, Endianness=little, Format=signed, Inversion=off, Startbit=50, Width_bits=12, Factor=1, Offset=0}
      | try
      | %
      | %Upgrade Information - standard BEGIN
      | new_color = 'blue';
      | new_ver = '0.19';
      | act_ver = get_param(gcb,'tt_iolib_version');
      | if not(strcmp(act_ver,new_ver))
      |     disp(['Upgrade block: ',gcb,char(10),'       Version: ',act_ver,' -> ',new_ver]);
      |     %switch - case for specific upgrade information e.g. additional parameter required 
      |     %Change appearance and version information
      |     set_param(gcb,'ForegroundColor',new_color);
      |     set_param(gcb,'tt_iolib_version',new_ver);
      | end
      | %Upgrade Information - standard END
      | catch
      | %Standard catch section BEGIN 
      | disp(' ');
      | disp('------------------------------------------------------------');
      | disp('An error occurred in a callback of the TTC580-BlockLib.');
      | disp(['Please check the parameters in the mask of ',gcb]);
      | disp('If you do not encounter any violations, then please '); 
      | disp('copy the following lines and report this to support@ttcontrol.com ');
      | disp('<< begin of error message dump >>');
      | disp(['Version of TTC580-BlockLib: ', get_param(gcb,'tt_iolib_version')]);
      | disp(get_param(gcb,'ttDescription'));
      | disp(gcb);
      | x=lasterror;disp(x.message);
      | disp(get_param(gcb,'MaskValues'));
      | disp(version);
      | disp(computer);
      | disp('<< end of error message dump >>');
      | disp('------------------------------------------------------------');
      | disp(' ');
      | %Standard catch section END
      | end
      mask help:
      | Block to prepare CAN-transmition at specified position within 64bit field.
      | For "Factor" and "Offset" the definition of Vector's CANdb applies:
      | [Physical value] = ( [Raw value] * [Factor] ) + [Offset]
      | with Raw value of a signal being the value as it is transmitted in the CAN-network.
      mask init:
      | %
      mask Help: web(which('IOLib500_utils.h'))
      mask TypeOptions Endianness: big | little
      mask Callback Endianness: %
      mask TypeOptions Format: unsigned | signed | real32
      mask Callback Format: %
      mask Callback Inversion: %
      mask Callback Startbit: %
      mask Callback Width_bits: %
      mask Callback Factor: %
      mask Callback Offset: %
  id_TX : Constant  Value=hex2dec('00001010')  OutDataTypeStr=uint32
  id_format_TX : Constant  OutDataTypeStr=Inherit: Inherit via back propagation
  length_TX : Constant  Value=8  OutDataTypeStr=Inherit: Inherit via back propagation
  ErrorCode : Outport
  wires:
  id_TX/1 -> IO_CAN_WriteMsg/5
  id_format_TX/1 -> IO_CAN_WriteMsg/4
  length_TX/1 -> IO_CAN_WriteMsg/3
  IO_CAN_ConfigMsg/2(handle) -> IO_CAN_WriteMsg/1
  IO_CAN_ConfigMsg/1(ErrorCode) -> Terminator5/1
  IO_CAN_WriteMsg/1 -> ErrorCode/1
  Test_u8_big/1 -> bit_packing1/1(Data_in)
  bit_packing1/1(Data_out) -> OR_TX/1
  Test_u16_big/1 -> bit_packing2/1(Data_in)
  bit_packing2/1(Data_out) -> OR_TX/2
  Test_i12_big/1 -> bit_packing3/1(Data_in)
  bit_packing3/1(Data_out) -> OR_TX/3
  Test_u8_little/1 -> bit_packing4/1(Data_in)
  bit_packing4/1(Data_out) -> OR_TX/4
  Test_i12_little/1 -> bit_packing5/1(Data_in)
  bit_packing5/1(Data_out) -> OR_TX/5
  OR_TX/1 -> IO_CAN_WriteMsg/2

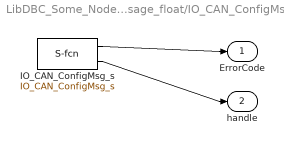
== system LibDBC_Some_Node_ch0_ORIGINAL/Rx_Message_float/IO_CAN_ConfigMsg ==
  IO_CAN_ConfigMsg_s : S-Function  FunctionName=IO_CAN_ConfigMsg_s  Parameters=SampleTime,channel,mode,id_format,id,ac_mask  SFunctionDeploymentMode=off  EnableBusSupport=off
  ErrorCode : Outport
  handle : Outport  Port=2
  wires:
  IO_CAN_ConfigMsg_s/2 -> handle/1
  IO_CAN_ConfigMsg_s/1 -> ErrorCode/1

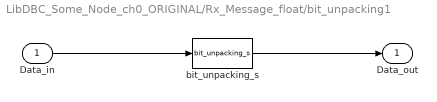
== system LibDBC_Some_Node_ch0_ORIGINAL/Rx_Message_float/bit_unpacking1 ==
  Data_in : Inport
  bit_unpacking_s : S-Function  FunctionName=bit_unpacking_s  Parameters=SampleTime,Endianness,Format,Inversion,Startbit,Width_bits,Factor,Offset  SFunctionDeploymentMode=off  EnableBusSupport=off
  Data_out : Outport
  wires:
  Data_in/1 -> bit_unpacking_s/1
  bit_unpacking_s/1 -> Data_out/1

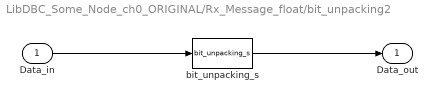
== system LibDBC_Some_Node_ch0_ORIGINAL/Rx_Message_float/bit_unpacking2 ==
  Data_in : Inport
  bit_unpacking_s : S-Function  FunctionName=bit_unpacking_s  Parameters=SampleTime,Endianness,Format,Inversion,Startbit,Width_bits,Factor,Offset  SFunctionDeploymentMode=off  EnableBusSupport=off
  Data_out : Outport
  wires:
  Data_in/1 -> bit_unpacking_s/1
  bit_unpacking_s/1 -> Data_out/1

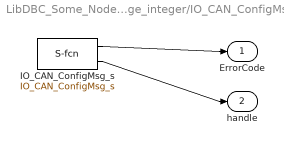
== system LibDBC_Some_Node_ch0_ORIGINAL/Rx_Message_integer/IO_CAN_ConfigMsg ==
  IO_CAN_ConfigMsg_s : S-Function  FunctionName=IO_CAN_ConfigMsg_s  Parameters=SampleTime,channel,mode,id_format,id,ac_mask  SFunctionDeploymentMode=off  EnableBusSupport=off
  ErrorCode : Outport
  handle : Outport  Port=2
  wires:
  IO_CAN_ConfigMsg_s/2 -> handle/1
  IO_CAN_ConfigMsg_s/1 -> ErrorCode/1

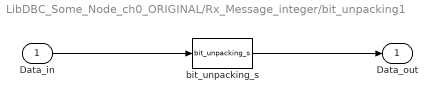
== system LibDBC_Some_Node_ch0_ORIGINAL/Rx_Message_integer/bit_unpacking1 ==
  Data_in : Inport
  bit_unpacking_s : S-Function  FunctionName=bit_unpacking_s  Parameters=SampleTime,Endianness,Format,Inversion,Startbit,Width_bits,Factor,Offset  SFunctionDeploymentMode=off  EnableBusSupport=off
  Data_out : Outport
  wires:
  Data_in/1 -> bit_unpacking_s/1
  bit_unpacking_s/1 -> Data_out/1

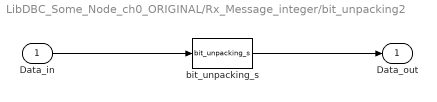
== system LibDBC_Some_Node_ch0_ORIGINAL/Rx_Message_integer/bit_unpacking2 ==
  Data_in : Inport
  bit_unpacking_s : S-Function  FunctionName=bit_unpacking_s  Parameters=SampleTime,Endianness,Format,Inversion,Startbit,Width_bits,Factor,Offset  SFunctionDeploymentMode=off  EnableBusSupport=off
  Data_out : Outport
  wires:
  Data_in/1 -> bit_unpacking_s/1
  bit_unpacking_s/1 -> Data_out/1

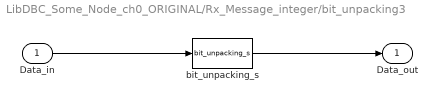
== system LibDBC_Some_Node_ch0_ORIGINAL/Rx_Message_integer/bit_unpacking3 ==
  Data_in : Inport
  bit_unpacking_s : S-Function  FunctionName=bit_unpacking_s  Parameters=SampleTime,Endianness,Format,Inversion,Startbit,Width_bits,Factor,Offset  SFunctionDeploymentMode=off  EnableBusSupport=off
  Data_out : Outport
  wires:
  Data_in/1 -> bit_unpacking_s/1
  bit_unpacking_s/1 -> Data_out/1

== system LibDBC_Some_Node_ch0_ORIGINAL/Rx_Message_integer/bit_unpacking4 ==
  Data_in : Inport
  bit_unpacking_s : S-Function  FunctionName=bit_unpacking_s  Parameters=SampleTime,Endianness,Format,Inversion,Startbit,Width_bits,Factor,Offset  SFunctionDeploymentMode=off  EnableBusSupport=off
  Data_out : Outport
  wires:
  Data_in/1 -> bit_unpacking_s/1
  bit_unpacking_s/1 -> Data_out/1

== system LibDBC_Some_Node_ch0_ORIGINAL/Rx_Message_integer/bit_unpacking5 ==
  Data_in : Inport
  bit_unpacking_s : S-Function  FunctionName=bit_unpacking_s  Parameters=SampleTime,Endianness,Format,Inversion,Startbit,Width_bits,Factor,Offset  SFunctionDeploymentMode=off  EnableBusSupport=off
  Data_out : Outport
  wires:
  Data_in/1 -> bit_unpacking_s/1
  bit_unpacking_s/1 -> Data_out/1

== system LibDBC_Some_Node_ch0_ORIGINAL/Test_Message_float/IO_CAN_ConfigMsg ==
  IO_CAN_ConfigMsg_s : S-Function  FunctionName=IO_CAN_ConfigMsg_s  Parameters=SampleTime,channel,mode,id_format,id,ac_mask  SFunctionDeploymentMode=off  EnableBusSupport=off
  ErrorCode : Outport
  handle : Outport  Port=2
  wires:
  IO_CAN_ConfigMsg_s/2 -> handle/1
  IO_CAN_ConfigMsg_s/1 -> ErrorCode/1

== system LibDBC_Some_Node_ch0_ORIGINAL/Test_Message_float/bit_packing1 ==
  Data_in : Inport
  bit_packing_s : S-Function  FunctionName=bit_packing_s  Parameters=SampleTime,Endianness,Format,Inversion,Startbit,Width_bits,Factor,Offset  SFunctionDeploymentMode=off  EnableBusSupport=off
  Data_out : Outport
  wires:
  Data_in/1 -> bit_packing_s/1
  bit_packing_s/1 -> Data_out/1

== system LibDBC_Some_Node_ch0_ORIGINAL/Test_Message_float/bit_packing2 ==
  Data_in : Inport
  bit_packing_s : S-Function  FunctionName=bit_packing_s  Parameters=SampleTime,Endianness,Format,Inversion,Startbit,Width_bits,Factor,Offset  SFunctionDeploymentMode=off  EnableBusSupport=off
  Data_out : Outport
  wires:
  Data_in/1 -> bit_packing_s/1
  bit_packing_s/1 -> Data_out/1

== system LibDBC_Some_Node_ch0_ORIGINAL/Test_Message_integer/IO_CAN_ConfigMsg ==
  IO_CAN_ConfigMsg_s : S-Function  FunctionName=IO_CAN_ConfigMsg_s  Parameters=SampleTime,channel,mode,id_format,id,ac_mask  SFunctionDeploymentMode=off  EnableBusSupport=off
  ErrorCode : Outport
  handle : Outport  Port=2
  wires:
  IO_CAN_ConfigMsg_s/2 -> handle/1
  IO_CAN_ConfigMsg_s/1 -> ErrorCode/1
